simulink model "NPC_1_modifs_openloop"  (R2013b)
settings: Solver=FixedStepDiscrete  SolverMode=SingleTasking  StartTime=0.0  StopTime=Inf  FixedStep=Tpas  MaxStep=100e-6  MinStep=50e-6  RelTol=1e-3
InitFcn:
  | Ts = 1e-6
values from neighbouring files (symbols this model uses):
  ech = 3000    [DCP_DCN_Para.m]
  Lch = 0.1    [DCP_DCN_Para.m]
  Lcoup = 1e-6    (= 1e-06)    [DCP_DCN_Para.m]
  Rch = 0.28    [DCP_DCN_Para.m]
  Tpas = 1e-5    (= 1e-05)    [DCP_DCN_Para.m]
  Vdc = 2500    [DCP_DCN_Para.m]
undefined symbols (not defined in the file or in its folder): DiscIntNeverNeededParam
libraries: powerlib x48, simulink x5, powerlib_meascontrol x3
settings Model: Creator=Daniel  LastModifiedBy=Daniel
settings SolverCC: InitialStep=50e-6  MaxConsecutiveMinStep=100000  AlgebraicLoopSolver=LineSearch
settings DataIOCC: SignalLoggingSaveFormat=ModelDataLogs
settings DebuggingCC: ArrayBoundsChecking=warning  AlgebraicLoopMsg=none  ArtificialAlgebraicLoopMsg=none  MultiTaskDSMMsg=warning  MultiTaskCondExecSysMsg=none  ParameterPrecisionLossMsg=none  UnconnectedInputMsg=none  UnconnectedOutputMsg=none  UnconnectedLineMsg=none  StateNameClashWarn=warning  StrictBusMsg=None
settings RTWCC: IncludeERTFirstTime=on

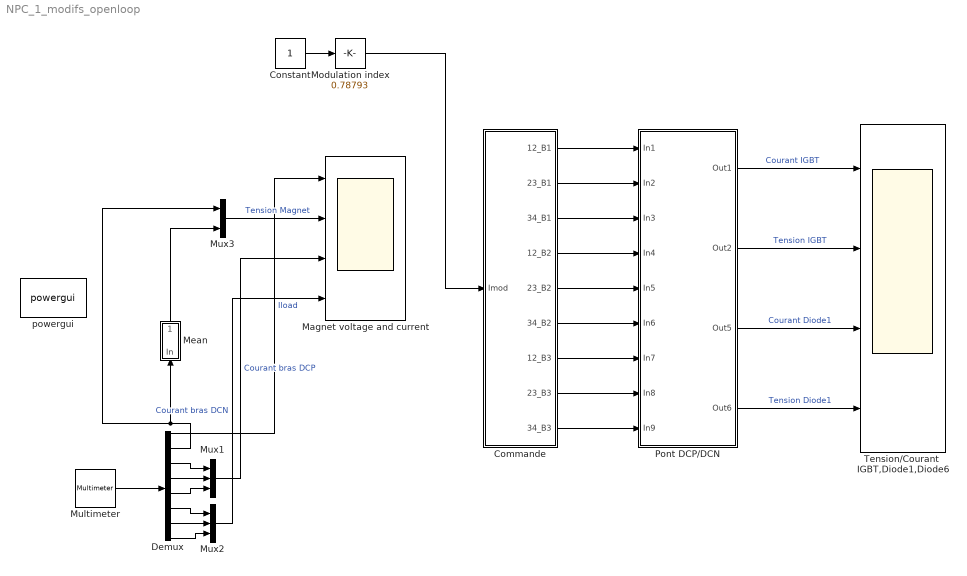
== system NPC_1_modifs_openloop ==
  Commande : Subsystem  SystemSampleTime=Ts
      settings: MinAlgLoopOccurrences=on
  Constant : Constant  SampleTime=Tpas
  Demux : Demux  Outputs=8
  Magnet voltage and current : Scope  NumInputPorts=4
      settings: YMin=-12500~-7500~-20000~-20000  YMax=15000~7500~20000~20000  MaxDataPoints=50000
  Mean : Subsystem
  "Modulation index " : simulink/Math Operations/Slider Gain  low=-0.95  gain=0.78793  high=0.95
  Multimeter : powerlib/Measurements/Multimeter  PhasorSimulation=off  OutputType=Complex  sel=[8 1 5 2 3 4 6 7]  L=8  Gain=[1 1 1 1 1 1 1 1]  yselected={'Ib: Pont DCP//DCN/Magnet','Ub: Pont DCP//DCN/Magnet','Ib: Pont DCP//DCN/DC2_B1','Ib: Pont DCP//DCN/DC1_B1','Ib: Pont DCP//DCN/DC1_B2','Ib: Pont DCP//DCN/DC1_B3','Ib: Pont DCP//DCN/DC2_B2','Ib: Pont DCP//DCN/DC2_B3'};  PSBOutputType=1  PSBequivalent=0  AxesSetting=[0,0.1,-100,100]  Display=0  SavedBlockNames=-11
  Mux1 : Mux  Inputs=3
  Mux2 : Mux  Inputs=3
  Mux3 : Mux  Inputs=2
  Pont DCP/DCN : Subsystem  SystemSampleTime=Ts
      settings: MinAlgLoopOccurrences=on
  Tension/Courant  IGBT,Diode1,Diode6 : Scope  NumInputPorts=4
      settings: YMin=-2500~-500~0~-3000  YMax=17500~3000~3500~500  SaveName=ScopeData2  MaxDataPoints=50000
  powergui : powerlib/powergui  Priority=1  SimulationMode=Discrete  SolverType=Tustin  SampleTime=Tpas  frequency=60  SPID=off  DisableSnubberDevices=off  DisableRonSwitches=off  DisableVfSwitches=off  SwTol=0  Interpol=off  DisplayEquations=off  frequencyindice=0  Pbase=100e6  ErrMax=1e-4  Iterations=50  UnitsV=kV  UnitsW=MW  FunctionMessages=off  echomessages=off  HookPort=off  EnableUseOfTLC=off  x0status=blocks  RestoreLinks=warning  ResistiveCurrentMeasurement=off  Frange=[0:2:500]  Ylog=off  Xlog=on  ShowGrid=off  save=off  variable=ZData  structure=ScopeData  ZoomFFT=off  StartTime=0.5  cycles=20  DisplayStyle=1  fundamental=1000  FreqAxis=off  MaxFrequency=10000  frequencyindicesteady=1  RmsSteady=1  display=off  Ts=0  methode=off
  wires:
  Multimeter/1 -> Demux/1
  Demux/2 -> Mean/1(In), Mux3/1
  Demux/3 -> Mux1/1
  Demux/4 -> Mux1/2
  Demux/5 -> Mux1/3
  Demux/6 -> Mux2/1
  Demux/7 -> Mux2/2
  Demux/8 -> Mux2/3
  Mux1/1 -> Magnet voltage and current/3  "Courant bras DCP"
  Mux2/1 -> Magnet voltage and current/4  "Courant bras DCN"
  Pont DCP/DCN/1(Out1) -> Tension/Courant  IGBT,Diode1,Diode6/1  "Courant IGBT"
  Pont DCP/DCN/2(Out2) -> Tension/Courant  IGBT,Diode1,Diode6/2  "Tension IGBT"
  Pont DCP/DCN/3(Out5) -> Tension/Courant  IGBT,Diode1,Diode6/3  "Courant Diode1"
  Pont DCP/DCN/4(Out6) -> Tension/Courant  IGBT,Diode1,Diode6/4  "Tension Diode1"
  Commande/1(12_B1) -> Pont DCP/DCN/1(In1)
  Commande/2(23_B1) -> Pont DCP/DCN/2(In2)
  Commande/3(34_B1) -> Pont DCP/DCN/3(In3)
  Commande/4(12_B2) -> Pont DCP/DCN/4(In4)
  Commande/5(23_B2) -> Pont DCP/DCN/5(In5)
  Commande/6("34_B2 ") -> Pont DCP/DCN/6(In6)
  Commande/7(12_B3) -> Pont DCP/DCN/7(In7)
  Commande/8(23_B3) -> Pont DCP/DCN/8(In8)
  Commande/9("34_B3 ") -> Pont DCP/DCN/9(In9)
  Mux3/1 -> Magnet voltage and current/2  "Tension Magnet"
  Mean/1(Out) -> Mux3/2
  Constant/1 -> "Modulation index "/1
  "Modulation index "/1 -> Commande/1(Imod)
  Demux/1 -> Magnet voltage and current/1  "Iload"

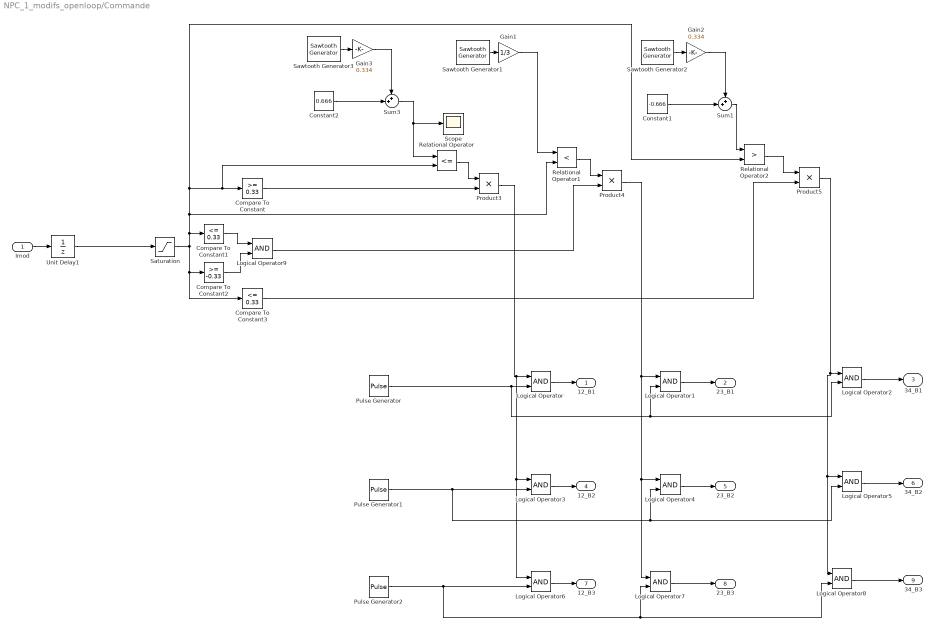
== system NPC_1_modifs_openloop/Commande ==
  Imod : Inport
  Compare To Constant : simulink/Logic and Bit Operations/Compare To Constant  relop=>=  const=0.33  OutDataTypeStr=boolean
  Compare To Constant1 : simulink/Logic and Bit Operations/Compare To Constant  relop=<=  const=0.33  OutDataTypeStr=boolean
  Compare To Constant2 : simulink/Logic and Bit Operations/Compare To Constant  relop=>=  const=-0.33  OutDataTypeStr=boolean
  Compare To Constant3 : simulink/Logic and Bit Operations/Compare To Constant  relop=<=  const=0.33  OutDataTypeStr=boolean
  Constant1 : Constant  Value=-0.666  SampleTime=Tpas
  Constant2 : Constant  Value=0.666  SampleTime=Tpas
  Gain1 : Gain  Gain=1/3  SampleTime=Tpas
  Gain2 : Gain  Gain=0.334  SampleTime=Tpas
  Gain3 : Gain  Gain=0.334  SampleTime=Tpas
  Logical Operator{,1..9} (10 alike) : Logic  AllPortsSameDT=off  OutDataTypeStr=boolean  SampleTime=Tpas
  Product3 : Product  SampleTime=Tpas
  Product4 : Product  SampleTime=Tpas
  Product5 : Product  SampleTime=Tpas
  Pulse Generator : DiscretePulseGenerator  Period=floor(3e-3/Tpas)  PulseWidth=floor(1e-3/Tpas)  SampleTime=Tpas
  Pulse Generator1 : DiscretePulseGenerator  Period=floor(3e-3/Tpas)  PulseWidth=floor(1e-3/Tpas)  PhaseDelay=floor(1e-3/Tpas)  SampleTime=Tpas
  Pulse Generator2 : DiscretePulseGenerator  Period=floor(3e-3/Tpas)  PulseWidth=floor(1e-3/Tpas)  PhaseDelay=floor(2e-3/Tpas)  SampleTime=Tpas
  Relational Operator : RelationalOperator  Operator=<=  OutDataTypeStr=boolean  SampleTime=Tpas
  Relational Operator1 : RelationalOperator  Operator=<  OutDataTypeStr=boolean  SampleTime=Tpas
  Relational Operator2 : RelationalOperator  Operator=>  OutDataTypeStr=boolean  SampleTime=Tpas
  Saturation : Saturate  UpperLimit=1  LowerLimit=-1
  Sawtooth Generator1 : powerlib_meascontrol/Pulse & Signal Generators/Sawtooth Generator  Freq=1e3  Phase=0  Ts=Tpas
  Sawtooth Generator2 : powerlib_meascontrol/Pulse & Signal Generators/Sawtooth Generator  Freq=1e3  Phase=0  Ts=Tpas
  Sawtooth Generator3 : powerlib_meascontrol/Pulse & Signal Generators/Sawtooth Generator  Freq=1e3  Phase=0  Ts=Tpas
  Scope : Scope
      settings: YMin=0.3  YMax=1
  Sum1 : Sum  Inputs=++|
  Sum3 : Sum  Inputs=++|
  Unit Delay1 : UnitDelay  SampleTime=-1
  12_B1 : Outport
  23_B1 : Outport  Port=2
  34_B1 : Outport  Port=3
  12_B2 : Outport  Port=4
  23_B2 : Outport  Port=5
  "34_B2 " : Outport  Port=6
  12_B3 : Outport  Port=7
  23_B3 : Outport  Port=8
  "34_B3 " : Outport  Port=9
  wires:
  Constant1/1 -> Sum1/2
  Sawtooth Generator1/1 -> Gain1/1
  Gain2/1 -> Sum1/1
  Sawtooth Generator2/1 -> Gain2/1
  Compare To Constant/1 -> Product3/2
  Compare To Constant3/1 -> Product5/2
  Saturation/1 -> Compare To Constant3/1, Compare To Constant2/1, Relational Operator2/2, Relational Operator/2, Compare To Constant/1, Relational Operator1/2, Compare To Constant1/1
  Gain1/1 -> Relational Operator1/1
  Sum1/1 -> Relational Operator2/1
  Pulse Generator/1 -> Logical Operator2/2, Logical Operator1/2, Logical Operator/2
  Pulse Generator1/1 -> Logical Operator3/2, Logical Operator5/2, Logical Operator4/2
  Pulse Generator2/1 -> Logical Operator8/2, Logical Operator7/2, Logical Operator6/2
  Logical Operator/1 -> 12_B1/1
  Logical Operator1/1 -> 23_B1/1
  Logical Operator2/1 -> 34_B1/1
  Logical Operator4/1 -> 23_B2/1
  Logical Operator7/1 -> 23_B3/1
  Logical Operator3/1 -> 12_B2/1
  Logical Operator6/1 -> 12_B3/1
  Logical Operator5/1 -> "34_B2 "/1
  Logical Operator8/1 -> "34_B3 "/1
  Sum3/1 -> Scope/1, Relational Operator/1
  Relational Operator/1 -> Product3/1
  Product3/1 -> Logical Operator6/1, Logical Operator3/1, Logical Operator/1
  Relational Operator1/1 -> Product4/1
  Product4/1 -> Logical Operator7/1, Logical Operator4/1, Logical Operator1/1
  Relational Operator2/1 -> Product5/1
  Product5/1 -> Logical Operator8/1, Logical Operator5/1, Logical Operator2/1
  Constant2/1 -> Sum3/2
  Gain3/1 -> Sum3/1
  Sawtooth Generator3/1 -> Gain3/1
  Compare To Constant1/1 -> Logical Operator9/1
  Compare To Constant2/1 -> Logical Operator9/2
  Logical Operator9/1 -> Product4/2
  Imod/1 -> Unit Delay1/1
  Unit Delay1/1 -> Saturation/1

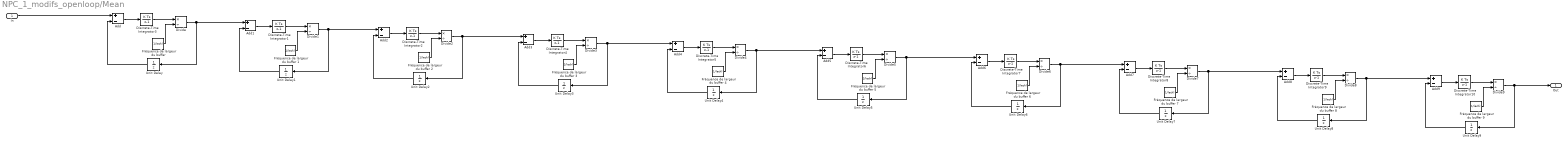
== system NPC_1_modifs_openloop/Mean ==
  In : Inport
  Add{,1..9} (10 alike) : Sum  Inputs=+-
  Discrete-Time Integrator{1..10} (10 alike) : DiscreteIntegrator  InitialConditionMode=State only (most efficient)  SampleTime=-1  ICPrevOutput=DiscIntNeverNeededParam  ICPrevScaledInput=DiscIntNeverNeededParam
  Divide{,1..9} (10 alike) : Product  Inputs=*/
  Fréquence de largeur du buffer {,1..9} (10 alike) : Constant  Value=1/(ech)
  Unit Delay{,1..9} (10 alike) : UnitDelay  SampleTime=-1
  Out : Outport
  wires:
  Add/1 -> Discrete-Time Integrator3/1
  "Fréquence de largeur du buffer "/1 -> Divide/2
  Discrete-Time Integrator3/1 -> Divide/1
  Unit Delay/1 -> Add/2
  Add1/1 -> Discrete-Time Integrator1/1
  Fréquence de largeur du buffer 1/1 -> Divide1/2
  Divide/1 -> Unit Delay/1, Add1/1
  Discrete-Time Integrator1/1 -> Divide1/1
  Unit Delay1/1 -> Add1/2
  Add2/1 -> Discrete-Time Integrator2/1
  Fréquence de largeur du buffer 2/1 -> Divide2/2
  Divide1/1 -> Unit Delay1/1, Add2/1
  Discrete-Time Integrator2/1 -> Divide2/1
  Unit Delay2/1 -> Add2/2
  Add3/1 -> Discrete-Time Integrator4/1
  Fréquence de largeur du buffer 3/1 -> Divide3/2
  Divide2/1 -> Unit Delay2/1, Add3/1
  Discrete-Time Integrator4/1 -> Divide3/1
  Unit Delay3/1 -> Add3/2
  In/1 -> Add/1
  Add4/1 -> Discrete-Time Integrator5/1
  Fréquence de largeur du buffer 4/1 -> Divide4/2
  Divide3/1 -> Add4/1, Unit Delay3/1
  Discrete-Time Integrator5/1 -> Divide4/1
  Unit Delay4/1 -> Add4/2
  Add5/1 -> Discrete-Time Integrator6/1
  Fréquence de largeur du buffer 5/1 -> Divide5/2
  Divide4/1 -> Add5/1, Unit Delay4/1
  Discrete-Time Integrator6/1 -> Divide5/1
  Unit Delay5/1 -> Add5/2
  Add6/1 -> Discrete-Time Integrator7/1
  Fréquence de largeur du buffer 6/1 -> Divide6/2
  Divide5/1 -> Add6/1, Unit Delay5/1
  Discrete-Time Integrator7/1 -> Divide6/1
  Unit Delay6/1 -> Add6/2
  Add7/1 -> Discrete-Time Integrator8/1
  Fréquence de largeur du buffer 7/1 -> Divide7/2
  Divide6/1 -> Add7/1, Unit Delay6/1
  Discrete-Time Integrator8/1 -> Divide7/1
  Unit Delay7/1 -> Add7/2
  Add8/1 -> Discrete-Time Integrator9/1
  Fréquence de largeur du buffer 8/1 -> Divide8/2
  Divide7/1 -> Unit Delay7/1, Add8/1
  Discrete-Time Integrator9/1 -> Divide8/1
  Unit Delay8/1 -> Add8/2
  Add9/1 -> Discrete-Time Integrator10/1
  Fréquence de largeur du buffer 9/1 -> Divide9/2
  Divide8/1 -> Add9/1, Unit Delay8/1
  Divide9/1 -> Out/1, Unit Delay9/1
  Discrete-Time Integrator10/1 -> Divide9/1
  Unit Delay9/1 -> Add9/2

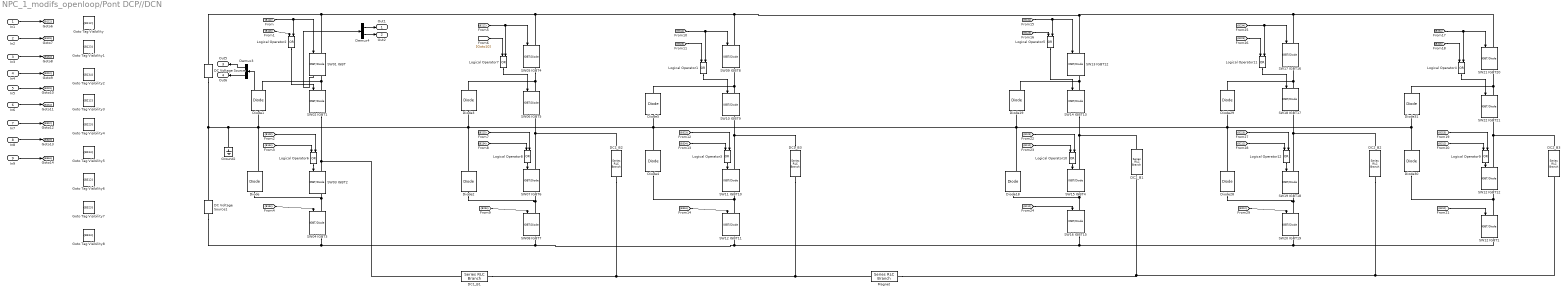
== system NPC_1_modifs_openloop/Pont DCP//DCN ==
  In1 : Inport
  In2 : Inport  Port=2
  In3 : Inport  Port=3
  In4 : Inport  Port=4
  In5 : Inport  Port=5
  In6 : Inport  Port=6
  In7 : Inport  Port=7
  In8 : Inport  Port=8
  In9 : Inport  Port=9
  DC Voltage Source : powerlib/Electrical Sources/DC Voltage Source  Amplitude=Vdc  Measurements=None
  DC Voltage Source1 : powerlib/Electrical Sources/DC Voltage Source  Amplitude=Vdc  Measurements=None
  DC1_B1 : powerlib/Elements/Series RLC Branch  LConnTagsString=__new0  RConnTagsString=__new0  BranchType=L  Resistance=0  Inductance=Lcoup  SetiL0=off  InitialCurrent=0  Capacitance=1e-6  Setx0=off  InitialVoltage=0  Measurements=Branch current
  DC1_B2 : powerlib/Elements/Series RLC Branch  LConnTagsString=__new0  RConnTagsString=__new0  BranchType=L  Resistance=0  Inductance=Lcoup  SetiL0=off  InitialCurrent=0  Capacitance=1e-6  Setx0=off  InitialVoltage=0  Measurements=Branch current
  DC1_B3 : powerlib/Elements/Series RLC Branch  LConnTagsString=__new0  RConnTagsString=__new0  BranchType=L  Resistance=0  Inductance=Lcoup  SetiL0=off  InitialCurrent=0  Capacitance=1e-6  Setx0=off  InitialVoltage=0  Measurements=Branch current
  DC2_B1 : powerlib/Elements/Series RLC Branch  LConnTagsString=__new0  RConnTagsString=__new0  BranchType=L  Resistance=0  Inductance=Lcoup  SetiL0=off  InitialCurrent=0  Capacitance=1e-6  Setx0=off  InitialVoltage=0  Measurements=Branch current
  DC2_B2 : powerlib/Elements/Series RLC Branch  LConnTagsString=__new0  RConnTagsString=__new0  BranchType=L  Resistance=0  Inductance=Lcoup  SetiL0=off  InitialCurrent=0  Capacitance=1e-6  Setx0=off  InitialVoltage=0  Measurements=Branch current
  DC2_B3 : powerlib/Elements/Series RLC Branch  LConnTagsString=__new0  RConnTagsString=__new0  BranchType=L  Resistance=0  Inductance=Lcoup  SetiL0=off  InitialCurrent=0  Capacitance=1e-6  Setx0=off  InitialVoltage=0  Measurements=Branch current
  Demux3 : Demux  Outputs=2
  Demux4 : Demux  Outputs=2
  Diode{,1,18..19} (4 alike) : powerlib/Power Electronics/Diode  Ron=0.001  Lon=0  Vf=0.8  IC=0  UseSnubber=off  Rs=1  Cs=inf  Measurements=on
  Diode{2..5,28..31} (8 alike) : powerlib/Power Electronics/Diode  Ron=0.001  Lon=0  Vf=0.8  IC=0  UseSnubber=off  Rs=1  Cs=inf  Measurements=off
  Goto Tag Visibility : GotoTagVisibility  GotoTag=B112
  Goto Tag Visibility1 : GotoTagVisibility  GotoTag=B123
  Goto Tag Visibility2 : GotoTagVisibility  GotoTag=B134
  Goto Tag Visibility3 : GotoTagVisibility  GotoTag=B212
  Goto Tag Visibility4 : GotoTagVisibility  GotoTag=B223
  Goto Tag Visibility5 : GotoTagVisibility  GotoTag=B234
  Goto Tag Visibility6 : GotoTagVisibility  GotoTag=B312
  Goto Tag Visibility7 : GotoTagVisibility  GotoTag=B323
  Goto Tag Visibility8 : GotoTagVisibility  GotoTag=B334
  Ground2 : powerlib/Elements/Ground  LConnTagsString=a
  Logical Operator{1..12} (12 alike) : Logic  Operator=OR  AllPortsSameDT=off  OutDataTypeStr=boolean
  Magnet : powerlib/Elements/Series RLC Branch  LConnTagsString=__new0  RConnTagsString=__new0  BranchType=RL  Resistance=Rch  Inductance=Lch  SetiL0=off  InitialCurrent=0  Capacitance=1e-6  Setx0=off  InitialVoltage=0  Measurements=Branch voltage and current
  SW01 IGBT : powerlib/Power Electronics/IGBT//Diode  Ron=Ron  Rs=Rs  Cs=Cs  Measurements=on
  SW02 IGBT1 : powerlib/Power Electronics/IGBT//Diode  Ron=Ron  Rs=Rs  Cs=Cs  Measurements=on
  SW03 IGBT2 : powerlib/Power Electronics/IGBT//Diode  Ron=Ron  Rs=Rs  Cs=Cs  Measurements=on
  SW04 IGBT3 : powerlib/Power Electronics/IGBT//Diode  Ron=Ron  Rs=Rs  Cs=Cs  Measurements=on
  SW05 IGBT4 : powerlib/Power Electronics/IGBT//Diode  Ron=Ron  Rs=Rs  Cs=Cs  Measurements=on
  SW06 IGBT5 : powerlib/Power Electronics/IGBT//Diode  Ron=Ron  Rs=Rs  Cs=Cs  Measurements=on
  SW07 IGBT6 : powerlib/Power Electronics/IGBT//Diode  Ron=Ron  Rs=Rs  Cs=Cs  Measurements=on
  SW08 IGBT7 : powerlib/Power Electronics/IGBT//Diode  Ron=Ron  Rs=Rs  Cs=Cs  Measurements=on
  SW09 IGBT8 : powerlib/Power Electronics/IGBT//Diode  Ron=Ron  Rs=Rs  Cs=Cs  Measurements=on
  SW10 IGBT9 : powerlib/Power Electronics/IGBT//Diode  Ron=Ron  Rs=Rs  Cs=Cs  Measurements=on
  SW11 IGBT10 : powerlib/Power Electronics/IGBT//Diode  Ron=Ron  Rs=Rs  Cs=Cs  Measurements=on
  SW12 IGBT1 : powerlib/Power Electronics/IGBT//Diode  Ron=Ron  Rs=Rs  Cs=Cs  Measurements=on
  SW12 IGBT11 : powerlib/Power Electronics/IGBT//Diode  Ron=Ron  Rs=Rs  Cs=Cs  Measurements=on
  SW12 IGBT12 : powerlib/Power Electronics/IGBT//Diode  Ron=Ron  Rs=Rs  Cs=Cs  Measurements=on
  SW13 IGBT12 : powerlib/Power Electronics/IGBT//Diode  Ron=Ron  Rs=Rs  Cs=Cs  Measurements=on
  SW14 IGBT13 : powerlib/Power Electronics/IGBT//Diode  Ron=Ron  Rs=Rs  Cs=Cs  Measurements=on
  SW15 IGBT4 : powerlib/Power Electronics/IGBT//Diode  Ron=Ron  Rs=Rs  Cs=Cs  Measurements=on
  SW16 IGBT15 : powerlib/Power Electronics/IGBT//Diode  Ron=Ron  Rs=Rs  Cs=Cs  Measurements=on
  SW17 IGBT16 : powerlib/Power Electronics/IGBT//Diode  Ron=Ron  Rs=Rs  Cs=Cs  Measurements=on
  SW18 IGBT17 : powerlib/Power Electronics/IGBT//Diode  Ron=Ron  Rs=Rs  Cs=Cs  Measurements=on
  SW19 IGBT18 : powerlib/Power Electronics/IGBT//Diode  Ron=Ron  Rs=Rs  Cs=Cs  Measurements=on
  SW20 IGBT19 : powerlib/Power Electronics/IGBT//Diode  Ron=Ron  Rs=Rs  Cs=Cs  Measurements=on
  SW21 IGBT20 : powerlib/Power Electronics/IGBT//Diode  Ron=Ron  Rs=Rs  Cs=Cs  Measurements=on
  SW22 IGBT21 : powerlib/Power Electronics/IGBT//Diode  Ron=Ron  Rs=Rs  Cs=Cs  Measurements=on
  Out1 : Outport
  Out2 : Outport  Port=2
  Out5 : Outport  Port=3
  Out6 : Outport  Port=4
  tag scope: B112=scoped, B123=scoped, B134=scoped, B212=scoped, B223=scoped, B234=scoped, B312=scoped, B323=scoped, B334=scoped
  wires:
  Logical Operator7/1 -> SW06 IGBT5/1
  Logical Operator3/1 -> SW11 IGBT10/1
  Logical Operator1/1 -> SW10 IGBT9/1
  [B323] -> Logical Operator3/2
  [B334] -> Logical Operator3/1
  [B123] -> Logical Operator10/2
  Logical Operator10/1 -> SW15 IGBT4/1
  [B223] -> Logical Operator12/2
  [B112] -> SW16 IGBT15/1
  [B212] -> SW20 IGBT19/1
  [B123] -> Logical Operator5/1
  [B112] -> Logical Operator10/1
  [B212] -> Logical Operator12/1
  Logical Operator6/1 -> SW03 IGBT2/1
  [B223] -> Logical Operator8/2
  [B112] -> SW01 IGBT/1, Logical Operator2/2
  [B323] -> Logical Operator1/1
  [B234] -> Logical Operator8/1
  Diode1/1 -> Demux3/1
  [B234] -> SW17 IGBT16/1, Logical Operator11/2
  [B334] -> SW21 IGBT20/1, Logical Operator4/2
  Logical Operator12/1 -> SW19 IGBT18/1
  [B323] -> Logical Operator9/2
  [B312] -> SW12 IGBT1/1
  Logical Operator4/1 -> SW22 IGBT21/1
  [B223] -> Logical Operator11/1
  Logical Operator5/1 -> SW14 IGBT13/1
  Logical Operator11/1 -> SW18 IGBT17/1
  Logical Operator9/1 -> SW12 IGBT12/1
  [B212] -> SW05 IGBT4/1, Logical Operator7/2
  Logical Operator2/1 -> SW02 IGBT1/1
  [B134] -> SW04 IGBT3/1
  [B323] -> Logical Operator4/1
  [B134] -> SW13 IGBT12/1, Logical Operator5/2
  [B123] -> Logical Operator6/2
  [B134] -> Logical Operator6/1
  [B312] -> SW09 IGBT8/1, Logical Operator1/2
  [B334] -> SW12 IGBT11/1
  [B234] -> SW08 IGBT7/1
  [B312] -> Logical Operator9/1
  [Goto10] -> Logical Operator7/1
  SW01 IGBT/1 -> Demux4/1
  Logical Operator8/1 -> SW07 IGBT6/1
  In1/1 -> [B112]
  In2/1 -> [B123]
  In3/1 -> [B134]
  In4/1 -> [B212]
  In5/1 -> [B223]
  In6/1 -> [B234]
  In7/1 -> [B312]
  In8/1 -> [B323]
  In9/1 -> [B334]
  Demux4/1 -> Out1/1
  Demux4/2 -> Out2/1
  Demux3/1 -> Out5/1
  Demux3/2 -> Out6/1
  [B123] -> Logical Operator2/1
  connections:
  Diode5/RConn1 -- SW09 IGBT8/RConn1 -- SW10 IGBT9/LConn1
  Diode29/RConn1 -- SW18 IGBT17/LConn1 -- SW17 IGBT16/RConn1
  Diode4/LConn1 -- SW12 IGBT11/LConn1 -- SW11 IGBT10/RConn1
  SW05 IGBT4/RConn1 -- SW06 IGBT5/LConn1 -- Diode3/RConn1
  Diode/LConn1 -- SW04 IGBT3/LConn1 -- SW03 IGBT2/RConn1
  DC1_B3/LConn1 -- SW11 IGBT10/LConn1 -- SW10 IGBT9/RConn1
  Diode19/LConn1 -- Diode4/RConn1 -- Diode5/LConn1 -- Diode2/RConn1 -- Diode3/LConn1 -- DC Voltage Source1/RConn1 -- DC Voltage Source/LConn1 -- Ground2/LConn1 -- Diode/RConn1 -- Diode1/LConn1 -- Diode18/RConn1 -- Diode28/RConn1 -- Diode29/LConn1 -- Diode30/RConn1 -- Diode31/LConn1
  DC1_B1/LConn1 -- SW02 IGBT1/RConn1 -- SW03 IGBT2/LConn1
  Diode30/LConn1 -- SW12 IGBT1/LConn1 -- SW12 IGBT12/RConn1
  DC2_B1/LConn1 -- SW14 IGBT13/RConn1 -- SW15 IGBT4/LConn1
  SW13 IGBT12/LConn1 -- SW09 IGBT8/LConn1 -- SW01 IGBT/LConn1 -- DC Voltage Source/RConn1 -- SW05 IGBT4/LConn1 -- SW21 IGBT20/LConn1 -- SW17 IGBT16/LConn1
  Diode18/LConn1 -- SW16 IGBT15/LConn1 -- SW15 IGBT4/RConn1
  DC2_B2/RConn1 -- DC2_B3/RConn1 -- Magnet/RConn1 -- DC2_B1/RConn1
  Diode31/RConn1 -- SW22 IGBT21/LConn1 -- SW21 IGBT20/RConn1
  Diode1/RConn1 -- SW02 IGBT1/LConn1 -- SW01 IGBT/RConn1
  Diode2/LConn1 -- SW08 IGBT7/LConn1 -- SW07 IGBT6/RConn1
  DC2_B2/LConn1 -- SW19 IGBT18/LConn1 -- SW18 IGBT17/RConn1
  Diode28/LConn1 -- SW20 IGBT19/LConn1 -- SW19 IGBT18/RConn1
  SW12 IGBT11/RConn1 -- SW12 IGBT1/RConn1 -- SW20 IGBT19/RConn1 -- SW16 IGBT15/RConn1 -- SW04 IGBT3/RConn1 -- DC Voltage Source1/LConn1 -- SW08 IGBT7/RConn1
  DC2_B3/LConn1 -- SW12 IGBT12/LConn1 -- SW22 IGBT21/RConn1
  DC1_B3/RConn1 -- Magnet/LConn1 -- DC1_B2/RConn1 -- DC1_B1/RConn1
  Diode19/RConn1 -- SW14 IGBT13/LConn1 -- SW13 IGBT12/RConn1
  DC1_B2/LConn1 -- SW07 IGBT6/LConn1 -- SW06 IGBT5/RConn1
